simulink model "Final_DC_MOTOR_Without_PID"  (R2021a)
settings: Solver=VariableStepAuto  StartTime=0.0  StopTime=35  MaxStep=0.001  RelTol=1e-3
values from neighbouring files (symbols this model uses):
  B = 0.015    [Project_reading_1.m]
  J = 0.0236    [Project_reading_1.m]
  k = 3    [Project_reading_1.m]
  Kt = 1.78    [Project_reading_1.m]
  L = 0.0063    [Project_reading_1.m]
  R = 2.1975    [Project_reading_1.m]
libraries: simulink_extras x2
settings Model: Creator=Panda  LastModifiedBy=Panda

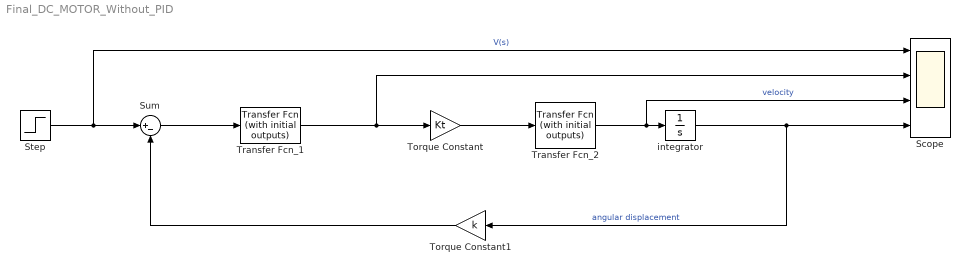
== system Final_DC_MOTOR_Without_PID ==
  Scope : Scope  NumInputPorts=4
  Step : Step  SampleTime=0
  Sum : Sum  Inputs=|+-
  Torque Constant : Gain  Gain=Kt
  Torque Constant1 : Gain  Gain=k
  "Transfer Fcn_1 " : simulink_extras/Additional Linear/Transfer Fcn (with initial outputs)  N=[1]  D="[L  R]"  Y0=.5  U0=0
  "Transfer Fcn_2 " : simulink_extras/Additional Linear/Transfer Fcn (with initial outputs)  N=[1]  D="[J  B]"  Y0=.5  U0=0
  integrator : Integrator
  wires:
  "Transfer Fcn_1 "/1 -> Scope/2, Torque Constant/1
  integrator/1 -> Torque Constant1/1, Scope/4  "angular displacement"
  Step/1 -> Scope/1, Sum/1  "V(s)"
  Sum/1 -> "Transfer Fcn_1 "/1
  Torque Constant/1 -> "Transfer Fcn_2 "/1
  Torque Constant1/1 -> Sum/2
  "Transfer Fcn_2 "/1 -> Scope/3, integrator/1  "velocity"
